simulink model "phi3_Autotrans_shift_expanded_breach"  (R2017a)
settings: Solver=ode5  StartTime=0.0  StopTime=tspan(end)  FixedStep=.01  RelTol=1e-3  AbsTol=1e-6
model workspace (MATLAB code in the model file):
  | load sldemo_autotrans_data; %load initial conditions and other necessary data
undefined symbols (not defined in the file or in its folder): downtab, emap, Iv, Kfactor, N20, Rfd, rload0, rload2, Rw, speedratio, Torkratio, uptab
Description:
  | Modeling an Automatic Transmission Controller
  | 
  | In this example, Simulink(R) is used to model an automotive drivetrain. Stateflow(R)
  | enhances the Simulink model with its representation of the transmission
  | control logic. Simulink provides a powerful environment for the modeling and
  | simulation of dynamic systems and processes. In many systems, though,
  | supervisory functions like changing modes or invoking new gain schedules must
  | respond to events that may occur and conditions that develop over time. As a
  | result, the environment requires a language capable of managing these multiple
  | modes and developing conditions. In the following example, Stateflow
  | demonstrates its strength in this capacity by performing the function of gear
  | selection in an automatic transmission. This function is combined with the
  | drivetrain dynamics in a natural and intuitive manner by incorporating a
  | Stateflow block in the Simulink block diagram.
settings Model: DataTypeOverride=Double  MinMaxOverflowLogging=ForceOff  SimulationMode=accelerator  ExtModeTrigMode=oneshot  ExtModeArmWhenConnect=off  ExtModeAutoUpdateStatusClock=off  Creator=The MathWorks Inc.  LastModifiedBy=nikhil
settings DataIOCC: ExternalInput=[t__, u__]  LoadExternalInput=on  SaveFormat=StructureWithTime  ReturnWorkspaceOutputs=on
settings OptimizationCC: BlockReduction=off  BooleanDataType=off  ExpressionDepthLimit=2147483647  InitFltsAndDblsToZero=on  LifeSpan=inf
settings DebuggingCC: SaveWithParameterizedLinksMsg=none  UnderspecifiedInitializationDetection=Classic  MergeDetectMultiDrivingBlocksExec=none  CheckExecutionContextPreStartOutputMsg=on  CheckExecutionContextRuntimeOutputMsg=on  SignalResolutionControl=TryResolveAllWithWarning  MultiTaskDSMMsg=warning  MultiTaskCondExecSysMsg=none  SigSpecEnsureSampleTimeMsg=none  IntegerOverflowMsg=none  FcnCallInpInsideContextMsg=warning  StateNameClashWarn=warning  SFUnexpectedBacktrackingDiag=warning  SFNoUnconditionalDefaultTransitionDiag=warning  SFExecutionAtInitializationDiag=none  IntegerSaturationMsg=none
settings HardwareCC: ProdBitPerPointer=32  ProdBitPerSizeT=32  ProdBitPerPtrDiffT=32  ProdLargestAtomicFloat=None  ProdIntDivRoundTo=Undefined  ProdEndianess=Unspecified  ProdWordSize=32  ProdHWDeviceType=32-bit Generic
settings ModelReferenceCC: PropagateSignalLabelsOutOfModel=off
settings SFSimCC: SFSimEcho=off
settings GRTTargetCC: TargetFcnLib=ansi_tfl_tmw.mat  TargetLangStandard=C89/C90 (ANSI)  GeneratePreprocessorConditionals=Disable all  CombineOutputUpdateFcns=off  GRTInterface=on
settings ConfigComp: CovEnable=on  RecordCoverage=on  CovMetricSettings=tr  CovHtmlReporting=on  CovSaveCumulativeToWorkspaceVar=on  CovSaveSingleToWorkspaceVar=on  CovModelRefEnable=on  CovExternalEMLEnable=off  CovSFcnEnable=off

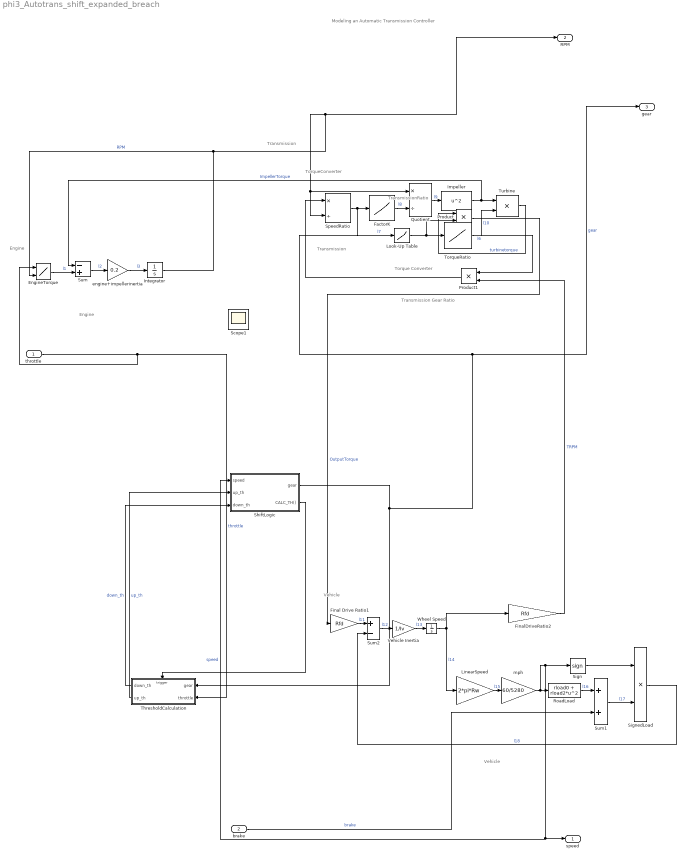
== system phi3_Autotrans_shift_expanded_breach ==
  note: TorqueConverter
  note: TransmissionRatio
  note: Vehicle
  note: Transmission
  note: Engine
  note: Modeling an Automatic Transmission Controller
  note: Engine
  note: Transmission
  note: Vehicle
  note: Transmission Gear Ratio
  note: Torque Converter
  throttle : Inport  Interpolate=off
  brake : Inport  Port=2  Interpolate=off
  EngineTorque : Lookup2D  RowIndex=thvec  ColumnIndex=nevec  Table=emap  InputSameDT=on
  FactorK : Lookup  InputValues=speedratio  Table=Kfactor  SaturateOnIntegerOverflow=on
  Final Drive Ratio1 : Gain  Gain=Rfd  SaturateOnIntegerOverflow=on  OutDataTypeStr=Inherit: Same as input  ParamDataTypeStr=Inherit: Same as input
  FinalDriveRatio2 : Gain  Gain=Rfd  SaturateOnIntegerOverflow=on  OutDataTypeStr=Inherit: Same as input  ParamDataTypeStr=Inherit: Same as input
  Impeller : Fcn  Expr=u^2
  Integrator : Integrator  InitialCondition=1000  LimitOutput=on  UpperSaturationLimit=6000  LowerSaturationLimit=600  ZeroCross=off
  LinearSpeed : Gain  Gain=2*pi*Rw  SaturateOnIntegerOverflow=on  OutDataTypeStr=Inherit: Same as input  ParamDataTypeStr=Inherit: Same as input
  Look-Up Table : Lookup  InputValues=[1 2 3 4]  Table=[2.393 1.450 1.000 0.677]  OutDataTypeStr=double  SaturateOnIntegerOverflow=on  LockScale=on
  Product : Product  SaturateOnIntegerOverflow=on  InputSameDT=on  OutDataTypeStr=Inherit: Same as first input
  Product1 : Product  SaturateOnIntegerOverflow=on  InputSameDT=on  OutDataTypeStr=Inherit: Same as first input
  Quotient : Product  Inputs=*/  SaturateOnIntegerOverflow=on  InputSameDT=on  OutDataTypeStr=Inherit: Same as first input
  RoadLoad : Fcn  Expr=rload0 + rload2*u^2
  ShiftLogic : Stateflow chart  TreatAsAtomicUnit=on
  Sign : Signum
  SignedLoad : Product  SaturateOnIntegerOverflow=on  InputSameDT=on  OutDataTypeStr=Inherit: Same as first input
  SpeedRatio : Product  Inputs=*/  SaturateOnIntegerOverflow=on  InputSameDT=on  OutDataTypeStr=Inherit: Same as first input
  Sum : Sum  Inputs=-+  SaturateOnIntegerOverflow=on  InputSameDT=on  OutDataTypeStr=Inherit: Same as first input
  Sum1 : Sum  SaturateOnIntegerOverflow=on  InputSameDT=on  OutDataTypeStr=Inherit: Same as first input
  Sum2 : Sum  Inputs=+-  SaturateOnIntegerOverflow=on  InputSameDT=on  OutDataTypeStr=Inherit: Same as first input
  ThresholdCalculation : Subsystem  TreatAsAtomicUnit=on
  TorqueRatio : Lookup  InputValues=speedratio  Table=Torkratio  SaturateOnIntegerOverflow=on
  Turbine : Product  SaturateOnIntegerOverflow=on  InputSameDT=on  OutDataTypeStr=Inherit: Same as first input
  Vehicle Inertia : Gain  Gain=1/Iv  SaturateOnIntegerOverflow=on  OutDataTypeStr=Inherit: Same as input  ParamDataTypeStr=Inherit: Same as input
  Wheel Speed : Integrator  InitialCondition=N20/Rfd  ZeroCross=off
  engine+impellerinertia : Gain  Gain=0.2  SaturateOnIntegerOverflow=on  OutDataTypeStr=Inherit: Same as input  ParamDataTypeStr=Inherit: Same as input
  mph : Gain  Gain=60/5280  SaturateOnIntegerOverflow=on  OutDataTypeStr=Inherit: Same as input  ParamDataTypeStr=Inherit: Same as input
  speed : Outport
  RPM : Outport  Port=2
  gear : Outport  Port=3
  Scope1 : Scope
  wires:
  Impeller/1 -> Sum/1, Turbine/1  "ImpellerTorque"
  Integrator/1 -> RPM/1, SpeedRatio/2, Quotient/1, EngineTorque/2  "RPM"
  FinalDriveRatio2/1 -> Product1/2  "TRPM"
  ThresholdCalculation/1(down_th) -> ShiftLogic/3(down_th)  "down_th"
  ThresholdCalculation/2(up_th) -> ShiftLogic/2(up_th)  "up_th"
  ShiftLogic/1(gear) -> ThresholdCalculation/1(gear), Look-Up Table/1, gear/1  "gear"
  ShiftLogic/2(CALC_TH()) -> ThresholdCalculation/Trigger
  mph/1 -> ShiftLogic/1(speed), speed/1, Sign/1, RoadLoad/1  "speed"
  throttle/1 -> EngineTorque/1, ThresholdCalculation/2(throttle)  "throttle"
  Product/1 -> Final Drive Ratio1/1  "OutputTorque"
  brake/1 -> Sum1/2  "brake"
  EngineTorque/1 -> Sum/2  "l1"
  engine+impellerinertia/1 -> Integrator/1  "l3"
  Sum/1 -> engine+impellerinertia/1  "l2"
  Turbine/1 -> Product/1  "turbinetorque"
  Final Drive Ratio1/1 -> Sum2/1  "l11"
  Wheel Speed/1 -> LinearSpeed/1, FinalDriveRatio2/1  "l14"
  LinearSpeed/1 -> mph/1  "l15"
  Sum2/1 -> Vehicle Inertia/1  "l12"
  Vehicle Inertia/1 -> Wheel Speed/1  "l13"
  SignedLoad/1 -> Sum2/2  "l18"
  Sign/1 -> SignedLoad/1
  RoadLoad/1 -> Sum1/1  "l16"
  Sum1/1 -> SignedLoad/2  "l17"
  Look-Up Table/1 -> Product1/1, Product/2  "l6"
  Product1/1 -> SpeedRatio/1
  SpeedRatio/1 -> TorqueRatio/1, FactorK/1  "l7"
  FactorK/1 -> Quotient/2  "l8"
  Quotient/1 -> Impeller/1  "l9"
  TorqueRatio/1 -> Turbine/2  "l10"

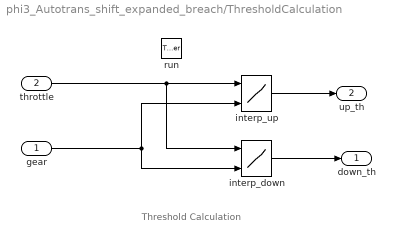
== system phi3_Autotrans_shift_expanded_breach/ThresholdCalculation ==
  note: Threshold Calculation
  gear : Inport
  throttle : Inport  Port=2
  run : TriggerPort  TriggerType=function-call  VariantControl=Variant  ZeroCross=off
  interp_down : Lookup2D  RowIndex=downth  ColumnIndex=[1:4]  Table=downtab  OutDataTypeStr=double
      settings: LockScale=on
  interp_up : Lookup2D  RowIndex=upth  ColumnIndex=[1:4]  Table=uptab  OutDataTypeStr=double
      settings: LockScale=on
  down_th : Outport
  up_th : Outport  Port=2
  wires:
  interp_up/1 -> up_th/1
  interp_down/1 -> down_th/1
  throttle/1 -> interp_up/1, interp_down/1
  gear/1 -> interp_up/2, interp_down/2

== stateflow chart phi3_Autotrans_shift_expanded_breach/ShiftLogic ==
  settings: updateMethod=DISCRETE  sampleTime=0.04
  state gear_state [parallel]
    settings: executionOrder=1
    state fourth
      entry:
      gear = 4;
    state third
      entry:
      gear = 3;
    state second
      entry:
      gear = 2;
    state first
      entry:
      gear = 1;
    (default) -> first
    second -> third [order 1] : UP
    first -> second : UP
    third -> fourth [order 1] : UP
    second -> first [order 2] : DOWN
    fourth -> third : DOWN
    third -> second [order 2] : DOWN
  state selection_state [parallel]
    during: CALC_TH;
    settings: executionOrder=2
    state steady_state
    state upshifting
    state downshifting
    (default) -> steady_state
    steady_state -> upshifting [order 1] : [speed > up_th]
    steady_state -> downshifting [order 2] : [speed < down_th]
    downshifting -> steady_state [order 2] : [speed > down_th]
    downshifting -> steady_state [order 1] : after(TWAIT,tick)
        | [speed <= down_th]
        | {gear_state.DOWN}
    upshifting -> steady_state [order 1] : after(TWAIT,tick)
        | [speed >= up_th]
        | {gear_state.UP}
    upshifting -> steady_state [order 2] : [speed < up_th]
  data: speed input double; gear output fixdt(0,8,5) [1..4]; TWAIT parameter fixdt(0,8,6); up_th input double; down_th input double
  events: DOWN local EITHER_EDGE_EVENT; UP local EITHER_EDGE_EVENT; CALC_TH output FUNCTION_CALL_EVENT
